simulink model "temp_rptgen_model"  (Simulink 3.00)
settings: Solver=FixedStepDiscrete  SolverMode=SingleTasking  StartTime=0.0  StopTime=10.0  RelTol=1e-3
Description:
  | This model is created by zslmethods/tempmodel as a dummy model.
settings Model: Tag=TempmodelCurrentModel  IntegerOverflowMsg=none  Creator=The MathWorks  LastModifiedBy=nikita

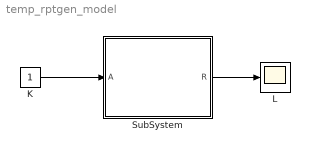
== system temp_rptgen_model ==
  K : Constant  Value=1
  L : Scope
      settings: TickLabels=on  TimeRange=auto  YMin=-5  YMax=5  SaveToWorkspace=off  SaveName=ScopeData  DataFormat=Matrix
  SubSystem : Subsystem  Tag=TempmodelCurrentSystem  Description=Selected by zslmethods/tempmodel as the current system
  wires:
  K/1 -> SubSystem/1(A)
  SubSystem/1(R) -> L/1

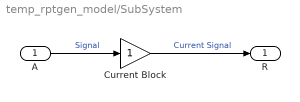
== system temp_rptgen_model/SubSystem ==
  A : Inport  Port=1  PortWidth=-1  SampleTime=-1  DataType=auto
      settings: SignalType=auto
  Current Block : Gain  Tag=TempmodelCurrentBlock  Description="This block is selected by zslmethods/tempmodel as the \"current\" block"  Gain=1  SaturateOnIntegerOverflow=on
  R : Outport  Port=1
  wires:
  A/1 -> Current Block/1  "Signal"
  Current Block/1 -> R/1  "Current Signal"
